simulink model "motor_controller_sim"  (R2019b)
settings: Solver=VariableStepAuto  StartTime=0.0  StopTime=t_max  RelTol=1e-3
values from neighbouring files (symbols this model uses):
  f = 0.00    (= 0)    [motor_controller_script.m]
  J = 0.5 * 10^(-4)    (= 5e-05)    [motor_controller_script.m]
  K_e = K_t    (= 0.004)    [motor_controller_script.m]
  K_t = 0.004    [motor_controller_script.m]
  L = 0.0    (= 0)    [motor_controller_script.m]
  M_b = 0.008    [motor_controller_script.m]
  P = 19 * K_e    (= 0.076)    [motor_controller_script.m]
  r = 500    [motor_controller_script.m]
  R = 2.0    (= 2)    [motor_controller_script.m]
settings Model: Creator=jpc  LastModifiedBy=jpc
settings DataIOCC: SaveOutput=off  SignalLogging=off  DSMLogging=off  ReturnWorkspaceOutputs=off  TimeSaveName=t_out

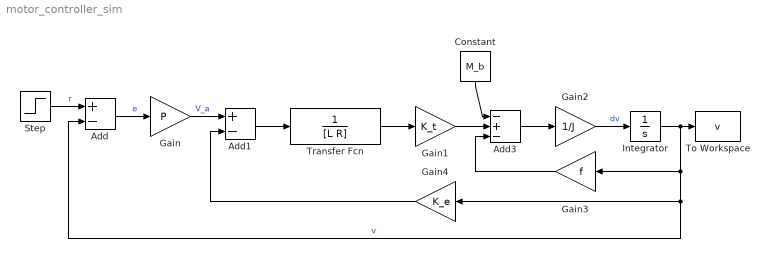
== system motor_controller_sim ==
  Add : Sum  Inputs=+-
  Add1 : Sum  Inputs=+-
  Add3 : Sum  Inputs=-+-
  Constant : Constant  Value=M_b
  Gain : Gain  Gain=P
  Gain1 : Gain  Gain=K_t
  Gain2 : Gain  Gain=1/J
  Gain3 : Gain  Gain=f
  Gain4 : Gain  Gain=K_e
  Integrator : Integrator
  Step : Step  Time=0  After=r  SampleTime=0
  To Workspace : ToWorkspace  VariableName=v  SampleTime=-1
      settings: Save2DSignal=2-D array (concatenate along first dimension)
  Transfer Fcn : TransferFcn  Denominator=[L R]
  wires:
  Add/1 -> Gain/1  "e"
  Gain/1 -> Add1/1  "V_a"
  Add1/1 -> Transfer Fcn/1
  Gain1/1 -> Add3/2
  Step/1 -> Add/1  "r"
  Transfer Fcn/1 -> Gain1/1
  Constant/1 -> Add3/1
  Add3/1 -> Gain2/1
  Gain2/1 -> Integrator/1  "dv"
  Gain3/1 -> Add3/3
  Gain4/1 -> Add1/2
  Integrator/1 -> Add/2, Gain4/1, Gain3/1, To Workspace/1  "v"
